simulink model "MCuC"  (R2025b)
settings: Solver=FixedStepDiscrete  StartTime=0.0  StopTime=10  RelTol=1e-3
undefined symbols (not defined in the file): BMS_Contactor_Command, MC_VSM_State, UC_State
libraries: simulink x8
settings Model: DataDictionary=rev3_data.sldd  Creator=mjmag  LastModifiedBy=diego
settings DataIOCC: ExternalInput=test_temp.getElement('Temp 1'),test_temp.getElement('Temp 2')  LoadExternalInput=on
settings OptimizationCC: DefaultParameterBehavior=Inlined  EnhancedBackFolding=on  PassReuseOutputArgsAs=Individual arguments  ZeroExternalMemoryAtStartup=off  ZeroInternalMemoryAtStartup=off  OptimizeBlockOrder=speed  DifferentSizesBufferReuse=on  OptimizationCustomize=off  EfficientTunableParamExpr=on
settings DebuggingCC: SolverPrmCheckMsg=warning  ParameterTunabilityLossMsg=error  StateNameClashWarn=warning
settings HardwareCC: ProdBitPerInt=16.0  ProdBitPerPointer=16.0  ProdBitPerSizeT=16.0  ProdBitPerPtrDiffT=16.0  ProdLargestAtomicFloat=None  ProdWordSize=16.0  ProdHWDeviceType=STMicroelectronics->ST10/Super10
settings SFSimCC: MATLABDynamicMemAlloc=off  SimTargetLang=C++  SimDLTargetLibrary=mkl-dnn
settings RTWCC: SystemTargetFile=ert.tlc  GenCodeOnly=on  TemplateMakefile=ert_default_tmf  BuildConfiguration=Faster Runs  PortableWordSizes=on  DataTypeReplacement=CDataTypesFixedWidth  TargetLang=C++  GPUComputeCapability=3.5  Description=Embedded Coder
settings CodeAppCC: ForceParamTrailComments=on  IgnoreCustomStorageClasses=off  OperatorAnnotations=on  SimulinkDataObjDesc=on  SFDataObjDesc=on  MATLABFcnDesc=on  InsertBlockDesc=on  StateflowObjectComments=on  InlinedPrmAccess=Macros
settings ERTTargetCC: RootIOFormat=Structure reference  ERTCustomFileTemplate=example_file_process.tlc  ERTFilePackagingFormat=Compact  SuppressUnreachableDefaultCases=off  IndentSize=4  MaxIdInt64=INT64_MAX  MinIdInt64=INT64_MIN  MaxIdUint64=UINT64_MAX  MaxIdInt32=INT32_MAX  MinIdInt32=INT32_MIN  MaxIdUint32=UINT32_MAX  MaxIdInt16=INT16_MAX  MinIdInt16=INT16_MIN  MaxIdUint16=UINT16_MAX  MaxIdInt8=INT8_MAX  MinIdInt8=INT8_MIN  MaxIdUint8=UINT8_MAX  DynamicArrayContainerType=coder::array  TargetLangStandard=C++11 (ISO)  GenerateSampleERTMain=on  CodeInterfacePackaging=C++ class  SubcomponentCodeInterfacePackaging=C++ class  PurelyIntegerCode=on  SupportNonFinite=off  SupportComplex=off  CastingMode=Standards  ArrayLayout=Row-major  ERTHeaderFileRootName=$R_Model$E  ERTSourceFileRootName=$R_Model$E

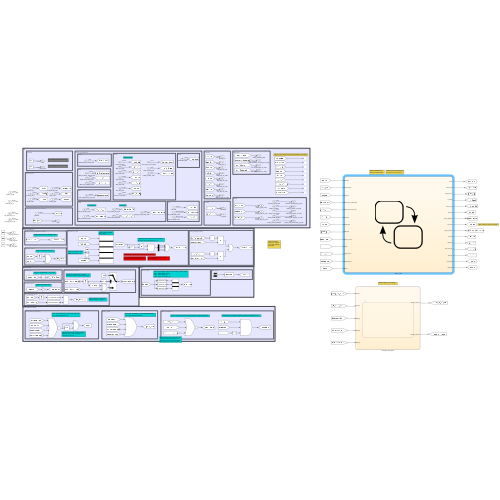
[thumbnail: Simulink's stored preview of the top-level diagram]
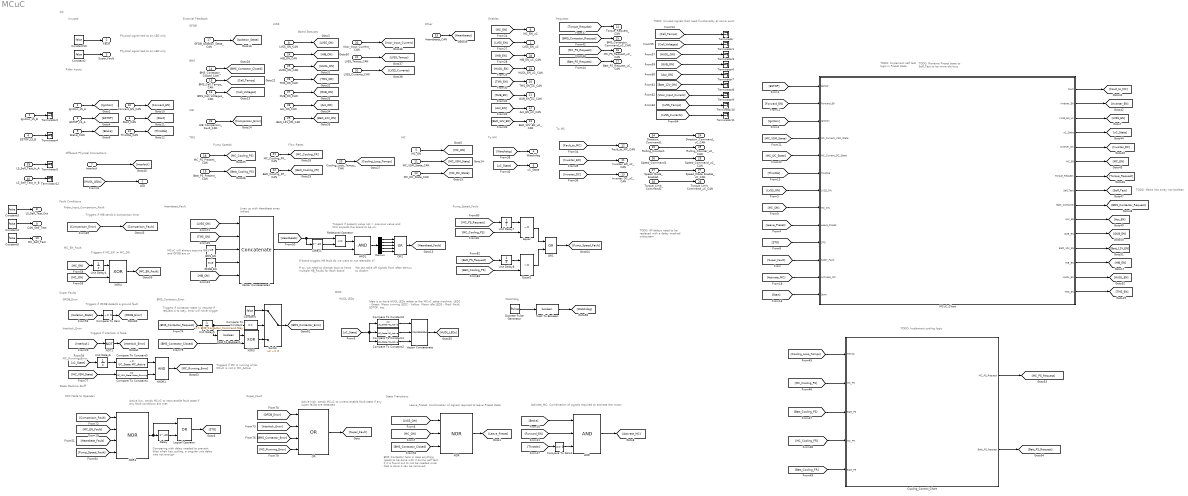
== system MCuC ==
  note: TODO: Rename Preset state to Self_Test to be more obvious
  note: MISC
  note: State Transitions
  note: GFDB_Error
  note: STO (Safe to Operate)
  note: MC_EN_Fault
  note: Watchdog
  note: Fault Conditions
  note: TODO: Unused signals that need functionality at some point
  note: State Machine Stuff
  note: Heartbeat_Fault
  note: I/O
  note: Other
  note: MC
  note: LVSS
  note: Pump Speeds
  note: GFDB
  note: External Feedback
  note: Offboard Physical Connections
  note: HUDL LEDs
  note: Rider Inputs
  note: If board triggers HB fault do we want to not reenable it?
  note: Lines up with Heartbeat array indices
  note: Active high, sends MCuC to unrecoverable fault state
      | if any super faults are detected
  note: Leave_Preset: Combination of signals required to leave Preset state
  note: Active low, sends MCuC to recoverable fault state if any fault conditions are met
  note: Physical signal tied to an LED only
  note: Idea is to have HUDL LEDs relate to the MCuC state machine.
      | LED1 - Green: Motor running
      | LED2 - Yellow: Motor idle
      | LED3 - Red: Fault, ESTOP, etc.
  note: Activate_MC: Combination of signals required to activate the motor
  note: Triggers if present value not > previous value and VCU expects the board to be on.
  note: TODO: Implement cooling logic
  note: Unused
  note: HIB
  note: BMS
  note: TMS
  note: Flow Rates
  note: Board Statuses
  note: Enables
  note: To MC
  note: To HM
  note: Requests
  note: MCuC will always assume
      | BMS and GFDB are on
  note: TODO: Make into array not boolean
  note: Comparing with delay needed to prevent blips when key cycling, a singular unit delay was not enough
  note: If so, we need to change logic to have multiple HB_Faults for each board
  note: Triggers if MC_EN != MC_ON
  note: Rider_Input_Comparison_Fault
  note: Triggers if HIB sends a comparison error
  note: Super Faults
  note: Super_Fault
  note: Triggers if GFDB detects a ground fault
  note: Triggers if Interlock is false
  note: Interlock_Error
  note: BMS_Contactor_Error
  note: Triggers if contactor state != request
      | If request is to stay, error will never trigger
  note: MC_Running_Error
  note: Triggers if MC is running while MCuC is not in MC_Active
  note: TODO: Implement self test logic in Preset state
  note: BMS_Contactor here in case anything needs to be done with it during self test, if it is found out to not be needed once that is done it can be removed
  note: We can take off signals from after demux to discern
  note: TODO: All delays need to be replaced with a delay masked subsystem
  note: Pump_Speed_Fault
  note: Physical signal tied to an LED only
  Ignition_LS_A : Inport  OutDataTypeStr=boolean
  Ignition_LS_B : Inport  Port=2  OutDataTypeStr=boolean
  ESTOP_LS_A : Inport  Port=3  OutDataTypeStr=boolean
  ESTOP_LS_B : Inport  Port=4  OutDataTypeStr=boolean
  MC_ON : Inport  Port=5  OutDataTypeStr=boolean
  Start_CAN : Inport  Port=6  OutDataTypeStr=boolean
  Interlock : Inport  Port=7  OutDataTypeStr=boolean
  LVSS_ON_CAN : Inport  Port=8  OutDataTypeStr=boolean
  Brake_CAN : Inport  Port=9  OutDataTypeStr=boolean
  Forward_EN_CAN : Inport  Port=10  OutDataTypeStr=boolean
  MC_VSM_State_CAN : Inport  Port=11  OutDataTypeStr=Enum: MC_VSM_State
  MC_DC_State_CAN : Inport  Port=12  OutDataTypeStr=Enum: MC_DC_State
  Throttle_CAN : Inport  Port=13  OutDataTypeStr=int16
  BMS_Contactor_Closed_CAN : Inport  Port=14  OutDataTypeStr=boolean
  BMS_Cell_Temps_CAN : Inport  Port=15  OutDataTypeStr=int32  PortDimensions=[1,45]
  BMS_Cell_Voltages_CAN : Inport  Port=16  OutDataTypeStr=int16  PortDimensions=[1,100]
  GFDB_Isolation_State_CAN : Inport  Port=17  OutDataTypeStr=uint8
  MC_PS_Present_CAN : Inport  Port=18  OutDataTypeStr=uint8
  Batt_PS_Present_CAN : Inport  Port=19  OutDataTypeStr=uint8
  Cooling_Loop_Temps_CAN : Inport  Port=20  OutDataTypeStr=int32  PortDimensions=[1,5]
  MC_Cooling_FR_CAN : Inport  Port=21  OutDataTypeStr=int16
  Batt_Cooling_FR_CAN : Inport  Port=22  OutDataTypeStr=int16
  HIB_Comparison_Fault_CAN : Inport  Port=23  OutDataTypeStr=boolean
  HIB_ON_CAN : Inport  Port=24  OutDataTypeStr=boolean
  HUDL_ON_CAN : Inport  Port=25  OutDataTypeStr=boolean
  TMS_ON_CAN : Inport  Port=26  OutDataTypeStr=boolean
  GUB_ON_CAN : Inport  Port=27  OutDataTypeStr=boolean
  Acc_ON_CAN : Inport  Port=28  OutDataTypeStr=boolean
  Batt_12V_ON_CAN : Inport  Port=29  OutDataTypeStr=boolean
  Vicor_Input_Current_CAN : Inport  Port=30  OutDataTypeStr=int16
  LVSS_Temps_CAN : Inport  Port=31  OutDataTypeStr=int32  PortDimensions=[1,6]
  LVSS_Currents_CAN : Inport  Port=32  OutDataTypeStr=int16  PortDimensions=[1,6]
  Heartbeats_CAN : Inport  Port=33  OutDataTypeStr=uint32  PortDimensions=[1,5]
  Direction_Command1 : Inport  Port=34  OutDataTypeStr=int16
  Rolling_Counter1 : Inport  Port=35  OutDataTypeStr=int16
  Speed_Command1 : Inport  Port=36  OutDataTypeStr=int16
  Speed_Mode_Enable1 : Inport  Port=37  OutDataTypeStr=int16
  Torque_Limit_Command1 : Inport  Port=38  OutDataTypeStr=int16
  LS_Self_Test_In_A : Inport  Port=39  OutDataTypeStr=boolean
  LS_Self_Test_In_B : Inport  Port=40  OutDataTypeStr=boolean
  AND : Logic  Inputs=3  IconShape=distinctive  AllPortsSameDT=off  OutDataTypeStr=boolean
  AND1 : Logic  IconShape=distinctive  AllPortsSameDT=off  OutDataTypeStr=boolean
  BMS_EN : Constant  Value=true  OutDataTypeStr=boolean
  Cast To Boolean : DataTypeConversion  OutDataTypeStr=boolean  SaturateOnIntegerOverflow=off  RndMeth=Floor
  Cast To Boolean1 : DataTypeConversion  OutDataTypeStr=boolean  SaturateOnIntegerOverflow=off  RndMeth=Floor
  Compare To Constant : simulink/Logic and Bit Operations/Compare To Constant  relop===  const=BMS_Contactor_Command.Stay  OutDataTypeStr=boolean
  Compare To Constant1 : simulink/Logic and Bit Operations/Compare To Constant  relop=<  const=UC_State.MC_Active  OutDataTypeStr=boolean
  Compare To Constant2 : simulink/Logic and Bit Operations/Compare To Constant  relop=>  const=UC_State.MC_Active  OutDataTypeStr=boolean
  Compare To Constant3 : simulink/Logic and Bit Operations/Compare To Constant  relop===  const=UC_State.MC_Active  OutDataTypeStr=boolean
  Compare To Constant4 : simulink/Logic and Bit Operations/Compare To Constant  relop===  const=MC_VSM_State.Motor_Running  OutDataTypeStr=boolean
  Compare To Constant5 : simulink/Logic and Bit Operations/Compare To Constant  relop=~=  const=UC_State.MC_Active  OutDataTypeStr=boolean
  Compare To Zero : simulink/Logic and Bit Operations/Compare To Zero  relop=~=  OutDataTypeStr=boolean
  Compare To Zero1 : simulink/Logic and Bit Operations/Compare To Zero  relop===  OutDataTypeStr=boolean
  Constant : Constant  Value=false  OutDataTypeStr=boolean
  Constant10 : Constant  Value=false  OutDataTypeStr=boolean
  Constant2 : Constant  Value=false  OutDataTypeStr=boolean
  Constant3 : Constant  Value=false
  Constant4 : Constant  Value=false
  Constant5 : Constant  Value=false
  Cooling_Control_Chart : Stateflow chart  TreatAsAtomicUnit=on
  Delay : Delay  DelayLength=20  InitialCondition=1
  Delay1 : Delay  DelayLength=10  InitialCondition=1
  Demux : Demux  Outputs=5
  Discrete Pulse Generator : DiscretePulseGenerator  Amplitude=true  Period=10  PulseWidth=5
  Equal : RelationalOperator  Operator=~=  OutDataTypeStr=boolean  RndMeth=Simplest  InputSameDT=off
  Equal1 : RelationalOperator  Operator=~=  OutDataTypeStr=boolean  RndMeth=Simplest  InputSameDT=off
  GFDB_EN : Constant  Value=true  OutDataTypeStr=boolean
  Logical Operator : Logic  Operator=OR  IconShape=distinctive  AllPortsSameDT=off  OutDataTypeStr=boolean
  MCuC_Chart : Stateflow chart  TreatAsAtomicUnit=on
      settings: PortSchema="{\"entries\":[{\"content\":{\"sides\":[{\"content\":{\"connectorIds\":[\"In1\",\"In2\",\"In3\",\"In5\",\"In6\",\"In7\",\"In8\",\"In9\",\"In4\",\"In10\",\"In11\",\"In12\",\"In13\"]},\"type\":\"ConnectorPlacement.EquallySpacedRectSide\",\"uuid\":\"cad206a9-8437-4e60-92a2-86fb9f7d0896\"},{\"content\":{\"connectorIds\":[\"Out1\",\"Out2\",\"Out3\",\"Out4\",\"Out5\",\"Out6\",\"Out7\",\"Out8\",\"Out9\",\"Out10\",\"Out11\",\"Out12\",\"Out13\",\"Out14\",\"Out15\"],\"side\":\"RIGHT\"},\"type\":\"ConnectorPlacement.EquallySpacedRectSide\",\"uuid\":\"f0e0577c-6f15-4024-8b2d-81740fdba28d\"},{\"content\":{\"side\":\"TOP\"},\"type\":\"ConnectorPlacement.EquallySpacedRectSide\",\"uuid\":\"9794c71a-d5bb-4555-9380-a4a6701a65fe\"}]},\"type\":\"ConnectorPlacement.EquallySpacedConnector\",\"uuid\":\"b2c715be-707d-43ed-bda8-ebb7411e45a6\"}],\"packageUris\":[\"http://schema.mathworks.com/mf0/Connector/R2020b\"],\"version\":\"1.0\"}"
  NOR : Logic  Operator=NOR  Inputs=3  IconShape=distinctive  AllPortsSameDT=off  OutDataTypeStr=boolean
  NOR1 : Logic  Operator=NOR  Inputs=4  IconShape=distinctive  AllPortsSameDT=off  OutDataTypeStr=boolean
  NOT1 : Logic  Operator=NOT  IconShape=distinctive  AllPortsSameDT=off  OutDataTypeStr=boolean
  NXOR1 : Logic  IconShape=distinctive  AllPortsSameDT=off  OutDataTypeStr=boolean
  OR : Logic  Operator=OR  Inputs=4  IconShape=distinctive  AllPortsSameDT=off  OutDataTypeStr=boolean
  OR1 : Logic  Operator=OR  IconShape=distinctive  AllPortsSameDT=off  OutDataTypeStr=boolean
  OR2 : Logic  Operator=OR  Inputs=5  IconShape=distinctive  AllPortsSameDT=off  OutDataTypeStr=boolean
  Relational Operator : RelationalOperator  Operator=<=  OutDataTypeStr=boolean  RndMeth=Simplest  InputSameDT=off
  Switch : Switch  Criteria=u2 ~= 0  SaturateOnIntegerOverflow=off  InputSameDT=off
  Terminator{,1..12} (13 alike) : Terminator
  Unit Delay4 : UnitDelay  SampleTime=-1  HasFrameUpgradeWarning=on
  Unit Delay5 : UnitDelay  InitialCondition=BMS_Contactor_Command.Open_Contactor  SampleTime=-1  HasFrameUpgradeWarning=on
  Unit Delay6 : UnitDelay  InitialCondition=UC_State.Preset  SampleTime=-1  HasFrameUpgradeWarning=on
  Unit Delay7 : UnitDelay  SampleTime=-1  HasFrameUpgradeWarning=on
  Unit Delay8 : UnitDelay  SampleTime=-1  HasFrameUpgradeWarning=on
  Vector Concatenate : Concatenate  NumInputs=3
  Vector Concatenate1 : Concatenate  NumInputs=5
  XOR3 : Logic  Operator=XOR  IconShape=distinctive  AllPortsSameDT=off  OutDataTypeStr=boolean
  XOR4 : Logic  Operator=XOR  IconShape=distinctive  AllPortsSameDT=off  OutDataTypeStr=boolean
  LVSS_EN_uC : Outport  OutDataTypeStr=boolean
  Fault : Outport  Port=2  OutDataTypeStr=boolean
  Super_Fault : Outport  Port=3  OutDataTypeStr=boolean
  Watchdog : Outport  Port=4  OutDataTypeStr=boolean
  uC_State : Outport  Port=5  OutDataTypeStr=Enum: UC_State
  MC_EN_uC : Outport  Port=6  OutDataTypeStr=boolean
  LED : Outport  Port=7  OutDataTypeStr=boolean  PortDimensions=[1,3]
  LS_Self_Test_Out : Outport  Port=8  OutDataTypeStr=boolean
  CAN_Self_Test : Outport  Port=9  OutDataTypeStr=boolean
  MC_Self_Test : Outport  Port=10  OutDataTypeStr=boolean
  Inverter_EN_uC_CAN : Outport  Port=11  OutDataTypeStr=boolean
  Fault_to_MC_CAN : Outport  Port=12  OutDataTypeStr=boolean
  Inverter_DC_uC_CAN : Outport  Port=13  OutDataTypeStr=boolean
  Torque_Request_CAN : Outport  Port=14  OutDataTypeStr=int16
  BMS_Contactor_Command_uC_CAN : Outport  Port=15  OutDataTypeStr=Enum: BMS_Contactor_Command
  MC_PS_Request_uC_CAN : Outport  Port=16  OutDataTypeStr=uint8
  Batt_PS_Request_uC_CAN : Outport  Port=17  OutDataTypeStr=uint8
  HIB_EN_uC_CAN : Outport  Port=18  OutDataTypeStr=boolean
  HUDL_EN_uC_CAN : Outport  Port=19  OutDataTypeStr=boolean
  TMS_EN_uC_CAN : Outport  Port=20  OutDataTypeStr=boolean
  GUB_EN_uC_CAN : Outport  Port=21  OutDataTypeStr=boolean
  Acc_EN_uC_CAN : Outport  Port=22  OutDataTypeStr=boolean
  Batt_12V_EN_uC_CAN : Outport  Port=23  OutDataTypeStr=boolean
  Direction_Command_uC_CAN : Outport  Port=24  OutDataTypeStr=int16
  Rolling_Counter_uC_CAN : Outport  Port=25  OutDataTypeStr=int16
  Speed_Command_uC_CAN : Outport  Port=26  OutDataTypeStr=int16
  Speed_Mode_Enable_uC_CAN : Outport  Port=27  OutDataTypeStr=int16
  Torque_Limit_Command_uC_CAN : Outport  Port=28  OutDataTypeStr=int16
  wires:
  TMS_ON_CAN/1 -> [TMS_ON]
  LVSS_Temps_CAN/1 -> [LVSS_Temps]
  HUDL_ON_CAN/1 -> [HUDL_ON]
  Vicor_Input_Current_CAN/1 -> [Vicor_Input_Current]
  HIB_ON_CAN/1 -> [HIB_ON]
  Batt_12V_ON_CAN/1 -> [Batt_12V_ON]
  LVSS_Currents_CAN/1 -> [LVSS_Currents]
  Acc_ON_CAN/1 -> [Acc_ON]
  GUB_ON_CAN/1 -> [GUB_ON]
  Constant10/1 -> Fault/1
  [Super_Fault] -> MCuC_Chart/11(Super_Fault)
  NOR/1 -> [Leave_Preset]
  LVSS_ON_CAN/1 -> [LVSS_ON]
  ESTOP_LS_A/1 -> [ESTOP]
  Ignition_LS_A/1 -> [Ignition]
  [ESTOP] -> MCuC_Chart/1(ESTOP)
  [Ignition] -> MCuC_Chart/3(Ignition)
  [LVSS_ON] -> MCuC_Chart/8(LVSS_ON)
  [Leave_Preset] -> MCuC_Chart/4(Leave_Preset)
  [LVSS_ON] -> NOR/1
  MC_ON/1 -> [MC_ON]
  [MC_ON] -> NOR/2
  [STO] -> MCuC_Chart/10(STO)
  [MC_ON] -> MCuC_Chart/9(MC_ON)
  MCuC_Chart/4(uC_State) -> [uC_State]
  [uC_State] -> Compare To Constant3/1, Compare To Constant2/1, Compare To Constant1/1
  AND/1 -> [Activate_MC]
  Brake_CAN/1 -> [Brake]
  Forward_EN_CAN/1 -> [Forward_EN]
  Start_CAN/1 -> [Start]
  Throttle_CAN/1 -> [Throttle]
  [Forward_EN] -> MCuC_Chart/2(Forward_EN)
  [Throttle] -> MCuC_Chart/7(Throttle)
  [Brake] -> AND/1
  [Forward_EN] -> AND/2
  [Throttle] -> Compare To Zero1/1
  Compare To Zero1/1 -> AND/3
  [MC_EN_Fault] -> NOR1/2
  [Activate_MC] -> MCuC_Chart/12(Activate_MC)
  Compare To Constant3/1 -> Vector Concatenate/1
  Compare To Constant1/1 -> Vector Concatenate/2
  Compare To Constant2/1 -> Vector Concatenate/3
  Delay1/1 -> Relational Operator/2
  AND1/1 -> Demux/1
  Relational Operator/1 -> AND1/1
  MCuC_Chart/15(TMS_EN) -> [TMS_EN]
  MCuC_Chart/3(LVSS_EN_uC) -> [LVSS_EN]
  BMS_EN/1 -> Vector Concatenate1/3
  GFDB_EN/1 -> Vector Concatenate1/4
  [HIB_ON] -> Vector Concatenate1/5
  Vector Concatenate1/1 -> AND1/2
  OR/1 -> [Super_Fault]
  Demux/1 -> OR2/1
  Demux/2 -> OR2/2
  Demux/3 -> OR2/3
  Demux/4 -> OR2/4
  Demux/5 -> OR2/5
  OR2/1 -> [Heartbeat_Fault]
  MC_VSM_State_CAN/1 -> [MC_VSM_State]
  MC_DC_State_CAN/1 -> [MC_DC_State]
  [MC_VSM_State] -> MCuC_Chart/5(MC_Current_VSM_State)
  [MC_DC_State] -> MCuC_Chart/6(MC_Current_DC_State)
  GFDB_Isolation_State_CAN/1 -> [Isolation_State]
  BMS_Contactor_Closed_CAN/1 -> [BMS_Contactor_Closed]
  BMS_Cell_Temps_CAN/1 -> [Cell_Temps]
  BMS_Cell_Voltages_CAN/1 -> [Cell_Voltages]
  HIB_Comparison_Fault_CAN/1 -> [Comparison_Error]
  MC_PS_Present_CAN/1 -> [MC_Cooling_PS]
  Batt_PS_Present_CAN/1 -> [Batt_Cooling_PS]
  Cooling_Loop_Temps_CAN/1 -> [Cooling_Loop_Temps]
  MC_Cooling_FR_CAN/1 -> [MC_Cooling_FR]
  Batt_Cooling_FR_CAN/1 -> [Batt_Cooling_FR]
  Heartbeats_CAN/1 -> [Heartbeats]
  Interlock/1 -> [Interlock]
  [MC_EN] -> MC_EN_uC/1
  [LVSS_EN] -> LVSS_EN_uC/1
  [HIB_EN] -> HIB_EN_uC_CAN/1
  [HUDL_EN] -> HUDL_EN_uC_CAN/1
  [TMS_EN] -> TMS_EN_uC_CAN/1
  [GUB_EN] -> GUB_EN_uC_CAN/1
  [Batt_12V_EN] -> Batt_12V_EN_uC_CAN/1
  [Acc_EN] -> Acc_EN_uC_CAN/1
  [Fault_to_MC] -> Fault_to_MC_CAN/1
  [Inverter_DC] -> Inverter_DC_uC_CAN/1
  [Inverter_EN] -> Inverter_EN_uC_CAN/1
  [Torque_Request] -> Torque_Request_CAN/1
  [uC_State] -> uC_State/1
  [Watchdog] -> Watchdog/1
  [HUDL_LEDs] -> LED/1
  [BMS_Contactor_Request] -> BMS_Contactor_Command_uC_CAN/1
  [MC_PS_Request] -> MC_PS_Request_uC_CAN/1
  [Batt_PS_Request] -> Batt_PS_Request_uC_CAN/1
  MCuC_Chart/1(Fault) -> [Fault_to_MC]
  MCuC_Chart/2(Inverter_EN) -> [Inverter_EN]
  MCuC_Chart/5(Inverter_DC) -> [Inverter_DC]
  MCuC_Chart/6(MC_EN) -> [MC_EN]
  MCuC_Chart/7(Torque_Request) -> [Torque_Request]
  MCuC_Chart/8(Self_Test) -> [Self_Test]
  MCuC_Chart/9(Batt_Contactor) -> [BMS_Contactor_Request]
  MCuC_Chart/10(Acc_EN) -> [Acc_EN]
  MCuC_Chart/11(GUB_EN) -> [GUB_EN]
  MCuC_Chart/12(Batt_12V_EN) -> [Batt_12V_EN]
  MCuC_Chart/13(HIB_EN) -> [HIB_EN]
  MCuC_Chart/14(HUDL_EN) -> [HUDL_EN]
  [Cooling_Loop_Temps] -> Cooling_Control_Chart/1(Temps)
  [MC_Cooling_PS] -> Cooling_Control_Chart/2(MC_PS)
  [Batt_Cooling_PS] -> Cooling_Control_Chart/3(Batt_PS)
  [MC_Cooling_FR] -> Cooling_Control_Chart/4(MC_FR)
  [Batt_Cooling_FR] -> Cooling_Control_Chart/5(Batt_FR)
  Cooling_Control_Chart/1(MC_PS_Request) -> [MC_PS_Request]
  Cooling_Control_Chart/2(Batt_PS_Request) -> [Batt_PS_Request]
  [Heartbeats] -> Delay1/1, Relational Operator/1
  [Comparison_Fault] -> NOR1/1
  [BMS_Contactor_Closed] -> NOR/3
  [Isolation_State] -> Compare To Zero/1
  [Cell_Temps] -> Terminator/1
  [Cell_Voltages] -> Terminator1/1
  [HUDL_ON] -> Terminator3/1
  [Batt_12V_ON] -> Terminator8/1
  [Acc_ON] -> Terminator7/1
  [GUB_ON] -> Terminator6/1
  [Vicor_Input_Current] -> Terminator9/1
  [LVSS_Currents] -> Terminator11/1
  [LVSS_Temps] -> Terminator10/1
  [LVSS_ON] -> Vector Concatenate1/1
  [TMS_ON] -> Vector Concatenate1/2
  Logical Operator/1 -> [STO]
  Delay/1 -> Logical Operator/2
  Discrete Pulse Generator/1 -> Cast To Boolean/1
  Cast To Boolean/1 -> [Watchdog]
  Unit Delay4/1 -> XOR4/1
  [MC_EN] -> Unit Delay4/1
  XOR4/1 -> [MC_EN_Fault]
  [Heartbeat_Fault] -> NOR1/3
  [MC_ON] -> XOR4/2
  [Comparison_Error] -> [Comparison_Fault]
  NOR1/1 -> Logical Operator/1, Delay/1
  Compare To Zero/1 -> [GFDB_Error]
  [GFDB_Error] -> OR/1
  [Interlock_Error] -> OR/2
  NOT1/1 -> [Interlock_Error]
  [Interlock] -> NOT1/1
  [BMS_Contactor_Request] -> Unit Delay5/1
  Compare To Constant/1 -> Switch/2
  Constant/1 -> Switch/1
  [BMS_Contactor_Closed] -> XOR3/2
  XOR3/1 -> Switch/3
  Unit Delay5/1 -> Cast To Boolean1/1, Compare To Constant/1
  Switch/1 -> [BMS_Contactor_Error]
  [BMS_Contactor_Error] -> OR/3
  Cast To Boolean1/1 -> XOR3/1
  [MC_VSM_State] -> Compare To Constant4/1
  [uC_State] -> Unit Delay6/1
  Unit Delay6/1 -> Compare To Constant5/1
  Compare To Constant5/1 -> NXOR1/1
  Compare To Constant4/1 -> NXOR1/2
  NXOR1/1 -> [MC_Running_Error]
  [MC_Running_Error] -> OR/4
  [Start] -> MCuC_Chart/13(Start)
  [MC_PS_Request] -> Unit Delay7/1
  [Batt_PS_Request] -> Unit Delay8/1
  Unit Delay7/1 -> Equal/1
  [MC_Cooling_PS] -> Equal/2
  [Batt_Cooling_PS] -> Equal1/2
  Unit Delay8/1 -> Equal1/1
  Equal/1 -> OR1/1
  Equal1/1 -> OR1/2
  OR1/1 -> [Pump_Speed_Fault]
  [Pump_Speed_Fault] -> NOR1/4
  Speed_Mode_Enable1/1 -> Speed_Mode_Enable_uC_CAN/1
  Direction_Command1/1 -> Direction_Command_uC_CAN/1
  Speed_Command1/1 -> Speed_Command_uC_CAN/1
  Torque_Limit_Command1/1 -> Torque_Limit_Command_uC_CAN/1
  Rolling_Counter1/1 -> Rolling_Counter_uC_CAN/1
  Vector Concatenate/1 -> [HUDL_LEDs]
  Constant2/1 -> Super_Fault/1
  Constant3/1 -> LS_Self_Test_Out/1
  Constant4/1 -> CAN_Self_Test/1
  Constant5/1 -> MC_Self_Test/1
  ESTOP_LS_B/1 -> Terminator4/1
  Ignition_LS_B/1 -> Terminator2/1
  LS_Self_Test_In_A/1 -> Terminator5/1
  LS_Self_Test_In_B/1 -> Terminator12/1

== stateflow chart MCuC/MCuC_Chart ==
  settings: executeAtInitialization=1
  state Logic [parallel]
    settings: executionOrder=1
    state LVSS_MC_Startup
      entry:
      MC_Uncharged = false;
      uC_State = UC_State.LVSS_MC_Startup;
      LVSS_EN_uC = true;
      MC_EN = true;
    state MC_Off
      entry:
      MC_EN = false;
      LVSS_EN_uC = false;
      uC_State = UC_State.MC_Off;
      MC_Uncharged = true;
      Inverter_EN = false;
    state LVSS_MC_Shutdown
      entry:
      uC_State = UC_State.LVSS_MC_Shutdown;
      LVSS_EN_uC = false;
      MC_EN = false;
    state Preset
      entry:
      uC_State = UC_State.Preset;
      Batt_Contactor = BMS_Contactor_Command.Open_Contactor;
      exit:
      Self_Test = false;
      state MC_ST
        entry:
        Self_Test = true;
        state MC_EN_ON
          entry:
          MC_EN = true;
        state MC_EN_OFF
          entry:
          MC_EN = false;
        (default) -> MC_EN_ON
        MC_EN_ON -> MC_EN_OFF : [MC_ON == true]
      (default) -> MC_ST
    state MC_Init
      entry:
      uC_State = UC_State.MC_Init;
      Batt_12V_EN = true;
      TMS_EN = true;
      HIB_EN = true;
      HUDL_EN = true;
      GUB_EN = true;
      Acc_EN = true;
    state MC_Discharging
      entry:
      uC_State = UC_State.MC_Discharging;
      exit:
      MC_Uncharged = true;
      Inverter_DC = false;
    state ESTOP
      entry:
      uC_State = UC_State.Estop;
      Batt_Contactor = BMS_Contactor_Command.Open_Contactor;
      LVSS_EN_uC = false;
      Activate_ESTOP = false;
    state Key_Cycle
      entry:
      uC_State = UC_State.Key_Cycle;
      Batt_Contactor = BMS_Contactor_Command.Close_Contactor;
    state Contactor_Closed
      entry:
      uC_State = UC_State.Contactor_Closed;
      Inverter_EN = false;
    state Contactor_Open
      entry:
      Inverter_EN = false;
      Inverter_DC = true;
      uC_State = UC_State.Contactor_Open;
      Acc_EN = false;
      GUB_EN = false;
      HUDL_EN = false;
      HIB_EN = false;
      TMS_EN = false;
      Batt_12V_EN = false;
    state Fault
      entry:
      uC_State = UC_State.Fault;
      Activate_Fault = false;
      Fault = true;
      Batt_Contactor = BMS_Contactor_Command.Stay;
      exit:
      Fault = false;
    state Super_Fault
      entry:
      uC_State = UC_State.Super_Fault;
      Batt_Contactor = BMS_Contactor_Command.Open_Contactor;
      Super_Super_Fault = true;
    state MC_Ready
      entry:
      uC_State = UC_State.MC_Ready;
      Inverter_EN = false;
    state MC_Active
      entry:
      Inverter_EN = true;
      uC_State = UC_State.MC_Active;
      Torque_Request = 0;
      during:
      Torque_Request = Throttle;
      end
      exit:
      Torque_Request = 0;
    LVSS_MC_Shutdown -> MC_Off : [MC_ON == false && LVSS_ON == false]
    (default) -> Preset
    MC_Off -> LVSS_MC_Startup : [Ignition == true]
    LVSS_MC_Startup -> MC_Init : [MC_ON == true && LVSS_ON == true]
    MC_Discharging -> LVSS_MC_Shutdown : [MC_Current_DC_State == MC_DC_State.Complete]
    Key_Cycle -> MC_Off : [Ignition == false]
    MC_EN_OFF -> Key_Cycle : [Leave_Preset == true]
    MC_Init -> Contactor_Open [order 1] : [Ignition == false]
    ESTOP -> Key_Cycle : [ESTOP == false]
    Logic -> ESTOP [order 3] : [ESTOP == true && MC_Uncharged == true && uC_State ~= UC_State.Preset]
    MC_Init -> Contactor_Closed [order 2] : [MC_Current_VSM_State == MC_VSM_State.Ready]
    Contactor_Open -> MC_Discharging : [MC_Current_DC_State ~= MC_DC_State.Disabled]
    Fault -> Key_Cycle : [STO == true]
    Logic -> Contactor_Open [order 2] : [Super_Fault == true && MC_Uncharged == false && Activate_Super_Fault == false]{Activate_Super_Fault = true;}
    Contactor_Closed -> Contactor_Open [order 1] : [Ignition == false]
    Logic -> Contactor_Open [order 4] : [ESTOP == true && MC_Uncharged == false && Activate_ESTOP == false]{Activate_ESTOP = true;}
    Logic -> Fault [order 5] : [STO == false && MC_Uncharged == true]
    Logic -> Contactor_Open [order 6] : [STO == false && MC_Uncharged == false && Activate_Fault == false]{Activate_Fault = true;}
    Contactor_Closed -> MC_Ready [order 2] : [Start == true]
    MC_Active -> Contactor_Open [order 2] : [Ignition == false]
    MC_Ready -> MC_Active : [Activate_MC == true]
    Logic -> Super_Fault [order 1] : [(Super_Fault == true && MC_Uncharged == true) || Super_Super_Fault == true]
    MC_Active -> MC_Ready [order 1] : [Forward_EN == false]
  data: Fault output =false; ESTOP input; Forward_EN input; Ignition input; Leave_Preset input; MC_Current_VSM_State input; Inverter_EN output =false; LVSS_EN_uC output =false; MC_Current_DC_State input; uC_State output =UC_State.MC_Off; MC_Uncharged local =true; Throttle input; Inverter_DC output =false; MC_EN output =false; LVSS_ON input; MC_ON input; Torque_Request output int16 =0; Self_Test output; STO input; Super_Fault input; Activate_ESTOP local =false; Activate_Fault local =false; Batt_Contactor output; Activate_MC input; Acc_EN output; GUB_EN output; Batt_12V_EN output; HIB_EN output; HUDL_EN output; TMS_EN output; Start input; Activate_Super_Fault local =false; Super_Super_Fault local =false

== stateflow chart MCuC/Cooling_Control_Chart ==
  state NOT_IMPLEMENTED
    entry:
    MC_PS_Request = MC_PS;
    Batt_PS_Request = Batt_PS;
    Temps;
    MC_FR;
    Batt_FR;
  (default) -> NOT_IMPLEMENTED
  data: Temps input; MC_PS input; Batt_PS input; MC_FR input; Batt_FR input; MC_PS_Request output; Batt_PS_Request output
